simulink model "wow_fail_prove"  (R2014b)
settings: Solver=FixedStepDiscrete  StartTime=0.0  StopTime=10.0  FixedStep=0.01  RelTol=1e-3
undefined symbols (not defined in the file): sldvsubsys
libraries: simulink x13, sldvlib x8
settings Model: ModifiedByFormat=Natasha  Creator=Natasha  LastModifiedBy=Natasha
settings DebuggingCC: UnderspecifiedInitializationDetection=Classic  MergeDetectMultiDrivingBlocksExec=none
settings ConfigComp: Description=Design Verifier Custom Configuration Component  DVMaxProcessTime=500000  DVMaxTestCaseSteps=500  DVTestSuiteOptimization=CombinedObjectives (Nonlinear Extended)  DVDetectActiveLogic=on

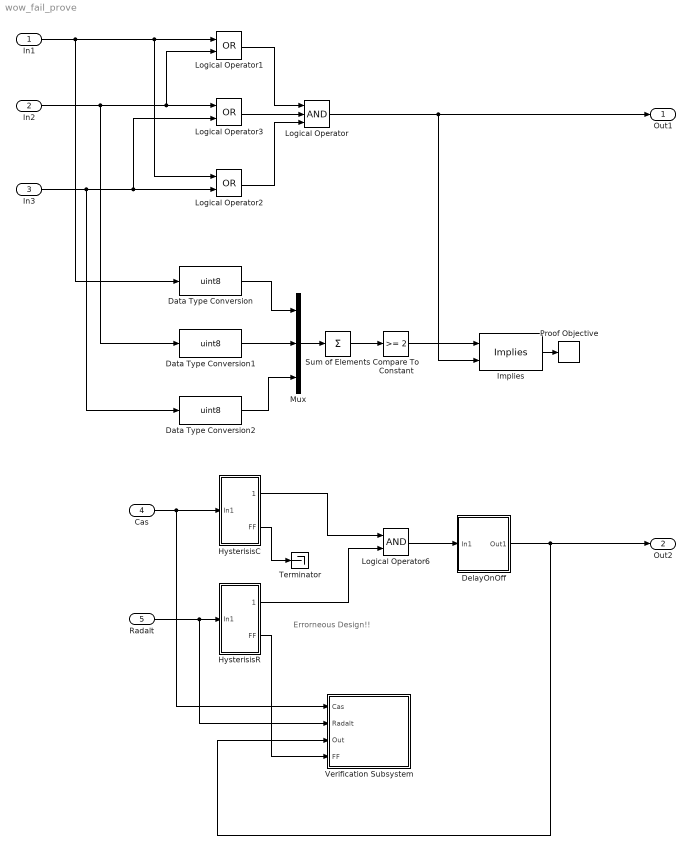
== system wow_fail_prove ==
  note: Errorneous Design!!
  In1 : Inport
  In2 : Inport  Port=2
  In3 : Inport  Port=3
  Cas : Inport  Port=4
  Radalt : Inport  Port=5
  Compare To Constant : simulink/Logic and Bit Operations/Compare To Constant  relop=>=  const=2  OutDataTypeStr=boolean
  Data Type Conversion : DataTypeConversion  OutDataTypeStr=uint8
  Data Type Conversion1 : DataTypeConversion  OutDataTypeStr=uint8
  Data Type Conversion2 : DataTypeConversion  OutDataTypeStr=uint8
  DelayOnOff : Subsystem
  HysterisisC : Subsystem
  HysterisisR : Subsystem
  Implies : sldvlib/Verification Utilities/Implies
  Logical Operator : Logic  Inputs=3  AllPortsSameDT=off  OutDataTypeStr=boolean
  Logical Operator1 : Logic  Operator=OR  AllPortsSameDT=off  OutDataTypeStr=boolean
  Logical Operator2 : Logic  Operator=OR  AllPortsSameDT=off  OutDataTypeStr=boolean
  Logical Operator3 : Logic  Operator=OR  AllPortsSameDT=off  OutDataTypeStr=boolean
  Logical Operator6 : Logic  AllPortsSameDT=off  OutDataTypeStr=boolean
  Mux : Mux  Inputs=3
  Proof Objective : sldvlib/Objectives and Constraints/Proof Objective  enabled=on  customAVTBlockType=Proof Objective  intervals=true  dispValues=on  outEnabled=off  enableStopSim=off
      settings: AttributesFormatString=%<intervals>
  Sum of Elements : Sum  Inputs=+
  Terminator : Terminator
  Verification Subsystem : Subsystem  Tag=VerificationSubsystem  DisableCoverage=on  LoadFcn=sldvsubsys('check')  TreatAsAtomicUnit=on  SimViewingDevice=on  mask(VerificationSubsystem){}
      mask init:
      | sldvsubsys('maskInit');
      settings: CopyFcn=sldvsubsys('copy');  OpenFcn=open_system(gcb,'force');
      settings: PreSaveFcn=|
      | set_param(gcb,'SimViewingDevice','on');
      | sldvsubsys('check');
      mask Help: helpview(fullfile(docroot,'toolbox','sldv','sldv.map'),'verificationsubsystem')
      mask Display: image(imread('sldvicon_versubsys.png','BackGroundColor',[1 1 1]),'center');
  Out1 : Outport
  Out2 : Outport  Port=2
  wires:
  Logical Operator/1 -> Implies/2, Out1/1
  Logical Operator1/1 -> Logical Operator/1
  In1/1 -> Logical Operator1/1, Logical Operator2/1, Data Type Conversion/1
  In2/1 -> Logical Operator3/1, Logical Operator1/2, Data Type Conversion1/1
  In3/1 -> Logical Operator2/2, Logical Operator3/2, Data Type Conversion2/1
  Logical Operator3/1 -> Logical Operator/2
  Logical Operator2/1 -> Logical Operator/3
  Data Type Conversion/1 -> Mux/1
  Data Type Conversion1/1 -> Mux/2
  Data Type Conversion2/1 -> Mux/3
  Mux/1 -> Sum of Elements/1
  Sum of Elements/1 -> Compare To Constant/1
  Compare To Constant/1 -> Implies/1
  Implies/1 -> Proof Objective/1
  Cas/1 -> Verification Subsystem/1(Cas), HysterisisC/1(In1)
  Radalt/1 -> Verification Subsystem/2(Radalt), HysterisisR/1(In1)
  HysterisisC/1(Out1) -> Logical Operator6/1
  HysterisisR/1(Out1) -> Logical Operator6/2
  HysterisisC/2(FF) -> Terminator/1
  HysterisisR/2(FF) -> Verification Subsystem/4(FF)
  Logical Operator6/1 -> DelayOnOff/1(In1)
  DelayOnOff/1(Out1) -> Verification Subsystem/3(Out), Out2/1

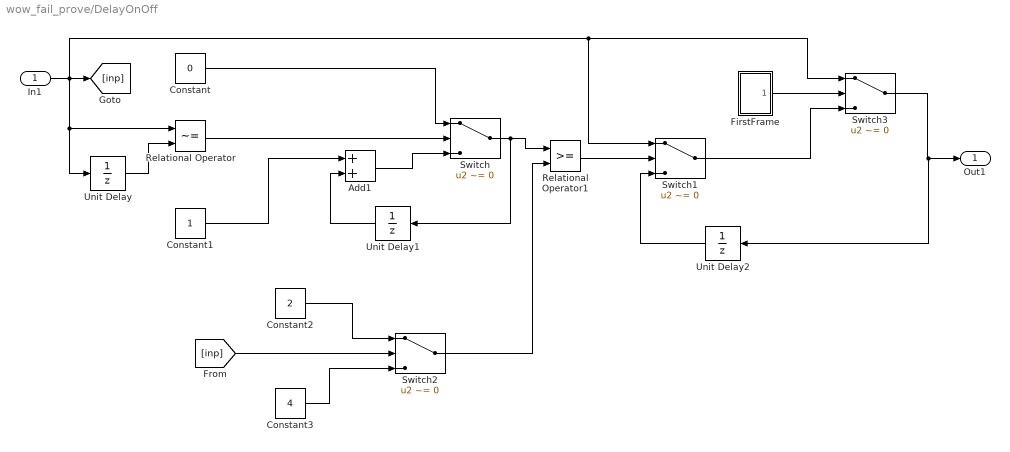
== system wow_fail_prove/DelayOnOff ==
  In1 : Inport
  Add1 : Sum
  Constant : Constant  Value=0
  Constant1 : Constant
  Constant2 : Constant  Value=2
  Constant3 : Constant  Value=4
  FirstFrame : Subsystem
  Relational Operator : RelationalOperator  Operator=~=  OutDataTypeStr=boolean
  Relational Operator1 : RelationalOperator  OutDataTypeStr=boolean
  Switch{,1..3} (4 alike) : Switch  Criteria=u2 ~= 0
  Unit Delay : UnitDelay  SampleTime=-1
  Unit Delay1 : UnitDelay  SampleTime=-1
  Unit Delay2 : UnitDelay  SampleTime=-1
  Out1 : Outport
  wires:
  Unit Delay1/1 -> Add1/2
  Constant2/1 -> Switch2/1
  Constant1/1 -> Add1/1
  Relational Operator/1 -> Switch/2
  Constant/1 -> Switch/1
  Unit Delay/1 -> Relational Operator/2
  Unit Delay2/1 -> Switch1/3
  Relational Operator1/1 -> Switch1/2
  Switch/1 -> Unit Delay1/1, Relational Operator1/1
  Constant3/1 -> Switch2/3
  Switch2/1 -> Relational Operator1/2
  Add1/1 -> Switch/3
  [inp] -> Switch2/2
  FirstFrame/1(Out1) -> Switch3/2
  In1/1 -> Switch3/1, Switch1/1, Unit Delay/1, Relational Operator/1, [inp]
  Switch1/1 -> Switch3/3
  Switch3/1 -> Unit Delay2/1, Out1/1

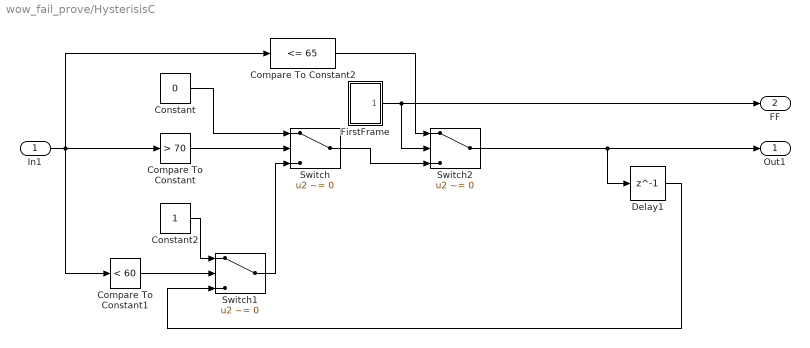
== system wow_fail_prove/HysterisisC ==
  In1 : Inport
  Compare To Constant : simulink/Logic and Bit Operations/Compare To Constant  relop=>  const=70  OutDataTypeStr=boolean
  Compare To Constant1 : simulink/Logic and Bit Operations/Compare To Constant  relop=<  const=60  OutDataTypeStr=boolean
  Compare To Constant2 : simulink/Logic and Bit Operations/Compare To Constant  relop=<=  const=65  OutDataTypeStr=boolean
  Constant : Constant  Value=0
  Constant2 : Constant
  Delay1 : Delay  DelayLength=1  InitialCondition=0
  FirstFrame : Subsystem
  Switch : Switch  Criteria=u2 ~= 0
  Switch1 : Switch  Criteria=u2 ~= 0
  Switch2 : Switch  Criteria=u2 ~= 0
  Out1 : Outport
  FF : Outport  Port=2
  wires:
  Compare To Constant2/1 -> Switch2/1
  Switch1/1 -> Switch/3
  Compare To Constant/1 -> Switch/2
  Delay1/1 -> Switch1/3
  In1/1 -> Compare To Constant/1, Compare To Constant1/1, Compare To Constant2/1
  Constant2/1 -> Switch1/1
  Switch/1 -> Switch2/3
  Compare To Constant1/1 -> Switch1/2
  Constant/1 -> Switch/1
  FirstFrame/1(Out1) -> FF/1, Switch2/2
  Switch2/1 -> Out1/1, Delay1/1

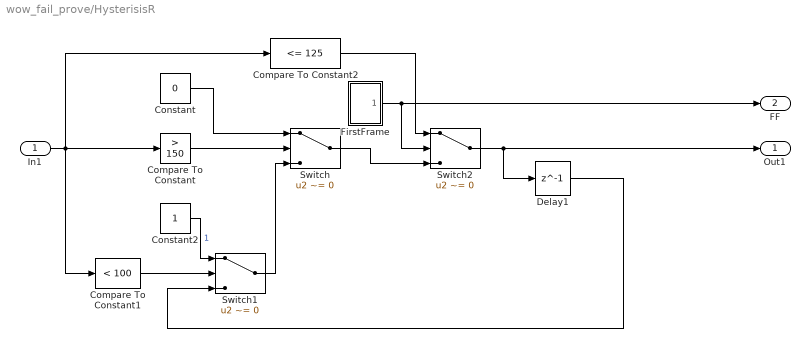
== system wow_fail_prove/HysterisisR ==
  In1 : Inport
  Compare To Constant : simulink/Logic and Bit Operations/Compare To Constant  relop=>  const=150  OutDataTypeStr=boolean
  Compare To Constant1 : simulink/Logic and Bit Operations/Compare To Constant  relop=<  const=100  OutDataTypeStr=boolean
  Compare To Constant2 : simulink/Logic and Bit Operations/Compare To Constant  relop=<=  const=125  OutDataTypeStr=boolean
  Constant : Constant  Value=0
  Constant2 : Constant
  Delay1 : Delay  DelayLength=1  InitialCondition=0
  FirstFrame : Subsystem
  Switch : Switch  Criteria=u2 ~= 0
  Switch1 : Switch  Criteria=u2 ~= 0
  Switch2 : Switch  Criteria=u2 ~= 0
  Out1 : Outport
  FF : Outport  Port=2
  wires:
  FirstFrame/1(Out1) -> Switch2/2, FF/1
  Constant/1 -> Switch/1
  Compare To Constant1/1 -> Switch1/2
  Switch/1 -> Switch2/3
  Constant2/1 -> Switch1/1  "1"
  In1/1 -> Compare To Constant2/1, Compare To Constant1/1, Compare To Constant/1
  Switch2/1 -> Delay1/1, Out1/1
  Delay1/1 -> Switch1/3
  Compare To Constant/1 -> Switch/2
  Switch1/1 -> Switch/3
  Compare To Constant2/1 -> Switch2/1

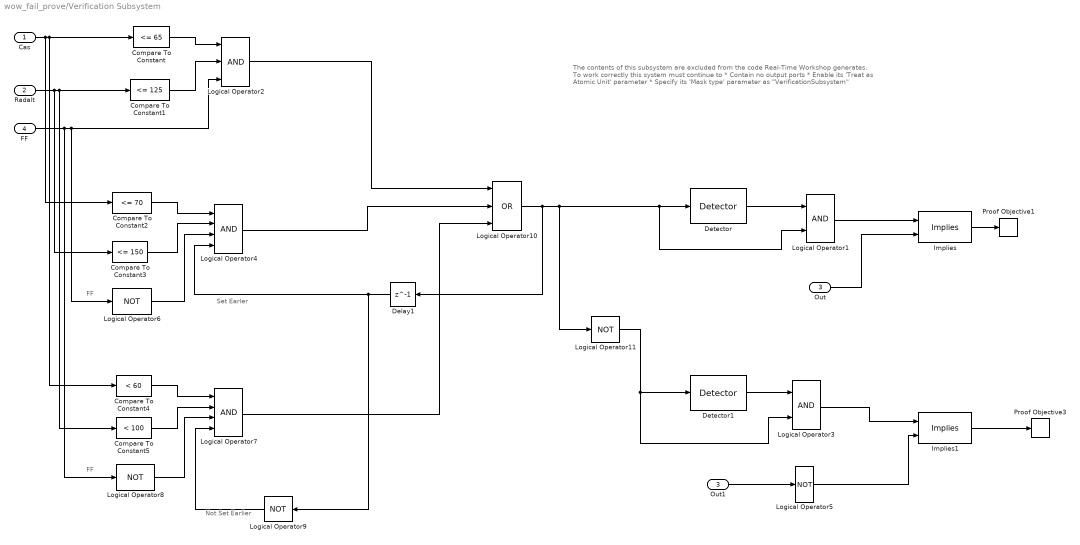
== system wow_fail_prove/Verification Subsystem ==
  note: FF
  note: FF
  note: Not Set Earlier
  note: Set Earler
  note: The contents of this subsystem are excluded from the code Real-Time
      | Workshop generates.
      |
      | To work correctly this system must continue to
      | * Contain no output ports
      | * Enable its 'Treat as Atomic Unit' parameter
      | * Specify its 'Mask type' parameter as "VerificationSubsystem"
  Cas : Inport
  Radalt : Inport  Port=2
  Out : Inport  Port=3
  FF : Inport  Port=4
  Compare To Constant : simulink/Logic and Bit Operations/Compare To Constant  relop=<=  const=65  OutDataTypeStr=boolean
  Compare To Constant1 : simulink/Logic and Bit Operations/Compare To Constant  relop=<=  const=125  OutDataTypeStr=boolean
  Compare To Constant2 : simulink/Logic and Bit Operations/Compare To Constant  relop=<=  const=70  OutDataTypeStr=boolean
  Compare To Constant3 : simulink/Logic and Bit Operations/Compare To Constant  relop=<=  const=150  OutDataTypeStr=boolean
  Compare To Constant4 : simulink/Logic and Bit Operations/Compare To Constant  relop=<  const=60  OutDataTypeStr=boolean
  Compare To Constant5 : simulink/Logic and Bit Operations/Compare To Constant  relop=<  const=100  OutDataTypeStr=boolean
  Delay1 : Delay  DelayLength=1  InitialCondition=0
  Detector : sldvlib/Temporal Operators/Detector  reset=off  typ=Synchronized  in_hold=3  delay=1  out_hold=3
  Detector1 : sldvlib/Temporal Operators/Detector  reset=off  typ=Synchronized  in_hold=5  delay=1  out_hold=3
  Implies : sldvlib/Verification Utilities/Implies
  Implies1 : sldvlib/Verification Utilities/Implies
  Logical Operator1 : Logic  AllPortsSameDT=off  OutDataTypeStr=boolean
  Logical Operator10 : Logic  Operator=OR  Inputs=3  AllPortsSameDT=off  OutDataTypeStr=boolean
  Logical Operator{5..6,8..9,11} (5 alike) : Logic  Operator=NOT  AllPortsSameDT=off  OutDataTypeStr=boolean
  Logical Operator2 : Logic  Inputs=3  AllPortsSameDT=off  OutDataTypeStr=boolean
  Logical Operator3 : Logic  AllPortsSameDT=off  OutDataTypeStr=boolean
  Logical Operator4 : Logic  Inputs=4  AllPortsSameDT=off  OutDataTypeStr=boolean
  Logical Operator7 : Logic  Inputs=4  AllPortsSameDT=off  OutDataTypeStr=boolean
  Out1 : InportShadow  Port=3
  Proof Objective1 : sldvlib/Objectives and Constraints/Proof Objective  enabled=on  customAVTBlockType=Proof Objective  intervals=true  dispValues=on  outEnabled=off  enableStopSim=on
      settings: AttributesFormatString=%<intervals>
  Proof Objective3 : sldvlib/Objectives and Constraints/Proof Objective  enabled=on  customAVTBlockType=Proof Objective  intervals=true  dispValues=on  outEnabled=off  enableStopSim=on
      settings: AttributesFormatString=%<intervals>
  wires:
  Out/1 -> Implies/2
  Compare To Constant/1 -> Logical Operator2/1
  Compare To Constant1/1 -> Logical Operator2/2
  Implies/1 -> Proof Objective1/1
  Logical Operator3/1 -> Implies1/1
  Detector1/1 -> Logical Operator3/1
  Compare To Constant2/1 -> Logical Operator4/1
  Compare To Constant3/1 -> Logical Operator4/2
  Implies1/1 -> Proof Objective3/1
  Logical Operator5/1 -> Implies1/2
  Out1/1 -> Logical Operator5/1
  Logical Operator6/1 -> Logical Operator4/3
  Delay1/1 -> Logical Operator9/1, Logical Operator4/4
  Cas/1 -> Compare To Constant2/1, Compare To Constant4/1, Compare To Constant/1
  Radalt/1 -> Compare To Constant3/1, Compare To Constant5/1, Compare To Constant1/1
  Compare To Constant4/1 -> Logical Operator7/1
  Compare To Constant5/1 -> Logical Operator7/2
  FF/1 -> Logical Operator8/1, Logical Operator6/1, Logical Operator2/3
  Logical Operator8/1 -> Logical Operator7/3
  Logical Operator9/1 -> Logical Operator7/4
  Logical Operator2/1 -> Logical Operator10/1
  Logical Operator4/1 -> Logical Operator10/2
  Logical Operator7/1 -> Logical Operator10/3
  Logical Operator10/1 -> Delay1/1, Logical Operator1/2, Detector/1, Logical Operator11/1
  Detector/1 -> Logical Operator1/1
  Logical Operator1/1 -> Implies/1
  Logical Operator11/1 -> Logical Operator3/2, Detector1/1

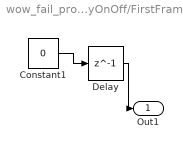
== system wow_fail_prove/DelayOnOff/FirstFrame ==
  Constant1 : Constant  Value=0
  Delay : Delay  DelayLength=1  InitialCondition=1
  Out1 : Outport
  wires:
  Constant1/1 -> Delay/1
  Delay/1 -> Out1/1

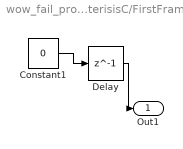
== system wow_fail_prove/HysterisisC/FirstFrame ==
  Constant1 : Constant  Value=0
  Delay : Delay  DelayLength=1  InitialCondition=1
  Out1 : Outport
  wires:
  Constant1/1 -> Delay/1
  Delay/1 -> Out1/1

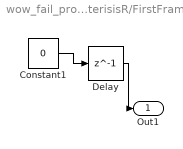
== system wow_fail_prove/HysterisisR/FirstFrame ==
  Constant1 : Constant  Value=0
  Delay : Delay  DelayLength=1  InitialCondition=1
  Out1 : Outport
  wires:
  Delay/1 -> Out1/1
  Constant1/1 -> Delay/1
